simulink model "RobotX_ss_acousticsSKIP_dock_odoa_ta_1021"  (R2014a)
settings: Solver=FixedStepDiscrete  StartTime=0.0  StopTime=inf  FixedStep=.25  RelTol=1e-3
undefined symbols (not defined in the file): Com1, Com2, Com3, Com4, DiscIntNeverNeededParam, standard
libraries: xpcseriallib x42, simulink x8, slrtlib x8, speedgoatlib x2, speedgoatlib_IO102 x1
(part 13 of 19)

== system RobotX_ss_acousticsSKIP_dock_odoa_ta_1021/Main FSM/ODOA/SLAM1/Models for prediction/Model39 ==
  X : Inport
  Y : Inport  Port=2
  Psi : Inport  Port=3
  Nav Messages : Inport  Port=4
  Bus Selector : BusSelector  OutputSignals=Velocity.u,Velocity.v,Velocity.r,Port.PtThrust,Port.PtAzimuth,Stbd.StThrust,Stbd.StAzimuth
  Data Store Read : DataStoreRead  DataStoreName=noiseLevel
  Demux : Demux  Outputs=3
  Discrete-Time Integrator1 : DiscreteIntegrator  SampleTime=-1  ICPrevOutput=DiscIntNeverNeededParam  ICPrevScaledInput=DiscIntNeverNeededParam
  Dynamic Model : MATLAB Function  TreatAsAtomicUnit=on
  Mux : Mux  Inputs=3
  Mux1 : Mux  Inputs=3
  Non-Holonomic Constraint : MATLAB Function  TreatAsAtomicUnit=on
  Port Thruster Model : MATLAB Function  TreatAsAtomicUnit=on
  Stbd Thruster Model : MATLAB Function  TreatAsAtomicUnit=on
  Sum : Sum  Inputs=|++|
  enabled : Constant
  move_part : MATLAB Function  TreatAsAtomicUnit=on
  NEyaw : Outport
  wires:
  Sum/1 -> Demux/1  "Forces"
  Bus Selector/2 -> Non-Holonomic Constraint/6(v), Dynamic Model/5(v)  "<v>"
  Bus Selector/1 -> Non-Holonomic Constraint/5(u), Dynamic Model/4(u)  "<u>"
  Psi/1 -> Non-Holonomic Constraint/8(psi), Dynamic Model/6(psi)
  Demux/2 -> Dynamic Model/2(F_sway)
  Demux/3 -> Dynamic Model/3(Torque)
  Demux/1 -> Dynamic Model/1(F_surge)
  Mux/1 -> Sum/2
  Stbd Thruster Model/1(F_surge) -> Mux/1
  Stbd Thruster Model/3(Torque) -> Mux/3
  Stbd Thruster Model/2(F_sway) -> Mux/2
  Mux1/1 -> Sum/1
  Port Thruster Model/2(F_sway) -> Mux1/2
  Port Thruster Model/1(F_surge) -> Mux1/1
  Port Thruster Model/3(Torque) -> Mux1/3
  Dynamic Model/1(surgeAccel) -> Non-Holonomic Constraint/2(surgeAccel)
  Dynamic Model/2(swayAccel) -> Non-Holonomic Constraint/3(swayAccel)
  Dynamic Model/3(yawAccel) -> Non-Holonomic Constraint/4(YawAccel)
  Y/1 -> Non-Holonomic Constraint/10(Y)
  X/1 -> Non-Holonomic Constraint/9(X)
  Bus Selector/3 -> Non-Holonomic Constraint/7(gyrz)  "<r>"
  Non-Holonomic Constraint/1(NEyaw) -> NEyaw/1
  enabled/1 -> Discrete-Time Integrator1/1
  Discrete-Time Integrator1/1 -> Non-Holonomic Constraint/1(time)
  Nav Messages/1 -> Bus Selector/1
  Bus Selector/4 -> move_part/1(PtThrust)  "<PtThrust>"
  Bus Selector/5 -> move_part/2(PtAzimuth)  "<PtAzimuth>"
  Bus Selector/7 -> move_part/4(StAzimuth)  "<StAzimuth>"
  Bus Selector/6 -> move_part/3(StThrust)  "<StThrust>"
  move_part/1(portMP) -> Port Thruster Model/1(portMP)
  move_part/2(portAzimuth) -> Port Thruster Model/2(portAzimuth)
  move_part/3(stbdMP) -> Stbd Thruster Model/1(stbdMP)
  move_part/4(stbdAzimuth) -> Stbd Thruster Model/2(stbdAzimuth)
  Data Store Read/1 -> move_part/5(noiseLevel)

== system RobotX_ss_acousticsSKIP_dock_odoa_ta_1021/Main FSM/ODOA/SLAM1/Models for prediction/Model4 ==
  X : Inport
  Y : Inport  Port=2
  Psi : Inport  Port=3
  Nav Messages : Inport  Port=4
  Bus Selector : BusSelector  OutputSignals=Velocity.u,Velocity.v,Velocity.r,Port.PtThrust,Port.PtAzimuth,Stbd.StThrust,Stbd.StAzimuth
  Data Store Read : DataStoreRead  DataStoreName=noiseLevel
  Demux : Demux  Outputs=3
  Discrete-Time Integrator1 : DiscreteIntegrator  SampleTime=-1  ICPrevOutput=DiscIntNeverNeededParam  ICPrevScaledInput=DiscIntNeverNeededParam
  Dynamic Model : MATLAB Function  TreatAsAtomicUnit=on
  Mux : Mux  Inputs=3
  Mux1 : Mux  Inputs=3
  Non-Holonomic Constraint : MATLAB Function  TreatAsAtomicUnit=on
  Port Thruster Model : MATLAB Function  TreatAsAtomicUnit=on
  Stbd Thruster Model : MATLAB Function  TreatAsAtomicUnit=on
  Sum : Sum  Inputs=|++|
  enabled : Constant
  move_part : MATLAB Function  TreatAsAtomicUnit=on
  NEyaw : Outport
  wires:
  Sum/1 -> Demux/1  "Forces"
  Bus Selector/2 -> Non-Holonomic Constraint/6(v), Dynamic Model/5(v)  "<v>"
  Bus Selector/1 -> Non-Holonomic Constraint/5(u), Dynamic Model/4(u)  "<u>"
  Psi/1 -> Non-Holonomic Constraint/8(psi), Dynamic Model/6(psi)
  Demux/2 -> Dynamic Model/2(F_sway)
  Demux/3 -> Dynamic Model/3(Torque)
  Demux/1 -> Dynamic Model/1(F_surge)
  Mux/1 -> Sum/2
  Stbd Thruster Model/1(F_surge) -> Mux/1
  Stbd Thruster Model/3(Torque) -> Mux/3
  Stbd Thruster Model/2(F_sway) -> Mux/2
  Mux1/1 -> Sum/1
  Port Thruster Model/2(F_sway) -> Mux1/2
  Port Thruster Model/1(F_surge) -> Mux1/1
  Port Thruster Model/3(Torque) -> Mux1/3
  Dynamic Model/1(surgeAccel) -> Non-Holonomic Constraint/2(surgeAccel)
  Dynamic Model/2(swayAccel) -> Non-Holonomic Constraint/3(swayAccel)
  Dynamic Model/3(yawAccel) -> Non-Holonomic Constraint/4(YawAccel)
  Y/1 -> Non-Holonomic Constraint/10(Y)
  X/1 -> Non-Holonomic Constraint/9(X)
  Bus Selector/3 -> Non-Holonomic Constraint/7(gyrz)  "<r>"
  Non-Holonomic Constraint/1(NEyaw) -> NEyaw/1
  enabled/1 -> Discrete-Time Integrator1/1
  Discrete-Time Integrator1/1 -> Non-Holonomic Constraint/1(time)
  Nav Messages/1 -> Bus Selector/1
  Bus Selector/4 -> move_part/1(PtThrust)  "<PtThrust>"
  Bus Selector/5 -> move_part/2(PtAzimuth)  "<PtAzimuth>"
  Bus Selector/7 -> move_part/4(StAzimuth)  "<StAzimuth>"
  Bus Selector/6 -> move_part/3(StThrust)  "<StThrust>"
  move_part/1(portMP) -> Port Thruster Model/1(portMP)
  move_part/2(portAzimuth) -> Port Thruster Model/2(portAzimuth)
  move_part/3(stbdMP) -> Stbd Thruster Model/1(stbdMP)
  move_part/4(stbdAzimuth) -> Stbd Thruster Model/2(stbdAzimuth)
  Data Store Read/1 -> move_part/5(noiseLevel)

== system RobotX_ss_acousticsSKIP_dock_odoa_ta_1021/Main FSM/ODOA/SLAM1/Models for prediction/Model40 ==
  X : Inport
  Y : Inport  Port=2
  Psi : Inport  Port=3
  Nav Messages : Inport  Port=4
  Bus Selector : BusSelector  OutputSignals=Velocity.u,Velocity.v,Velocity.r,Port.PtThrust,Port.PtAzimuth,Stbd.StThrust,Stbd.StAzimuth
  Data Store Read : DataStoreRead  DataStoreName=noiseLevel
  Demux : Demux  Outputs=3
  Discrete-Time Integrator1 : DiscreteIntegrator  SampleTime=-1  ICPrevOutput=DiscIntNeverNeededParam  ICPrevScaledInput=DiscIntNeverNeededParam
  Dynamic Model : MATLAB Function  TreatAsAtomicUnit=on
  Mux : Mux  Inputs=3
  Mux1 : Mux  Inputs=3
  Non-Holonomic Constraint : MATLAB Function  TreatAsAtomicUnit=on
  Port Thruster Model : MATLAB Function  TreatAsAtomicUnit=on
  Stbd Thruster Model : MATLAB Function  TreatAsAtomicUnit=on
  Sum : Sum  Inputs=|++|
  enabled : Constant
  move_part : MATLAB Function  TreatAsAtomicUnit=on
  NEyaw : Outport
  wires:
  Sum/1 -> Demux/1  "Forces"
  Bus Selector/2 -> Non-Holonomic Constraint/6(v), Dynamic Model/5(v)  "<v>"
  Bus Selector/1 -> Non-Holonomic Constraint/5(u), Dynamic Model/4(u)  "<u>"
  Psi/1 -> Non-Holonomic Constraint/8(psi), Dynamic Model/6(psi)
  Demux/2 -> Dynamic Model/2(F_sway)
  Demux/3 -> Dynamic Model/3(Torque)
  Demux/1 -> Dynamic Model/1(F_surge)
  Mux/1 -> Sum/2
  Stbd Thruster Model/1(F_surge) -> Mux/1
  Stbd Thruster Model/3(Torque) -> Mux/3
  Stbd Thruster Model/2(F_sway) -> Mux/2
  Mux1/1 -> Sum/1
  Port Thruster Model/2(F_sway) -> Mux1/2
  Port Thruster Model/1(F_surge) -> Mux1/1
  Port Thruster Model/3(Torque) -> Mux1/3
  Dynamic Model/1(surgeAccel) -> Non-Holonomic Constraint/2(surgeAccel)
  Dynamic Model/2(swayAccel) -> Non-Holonomic Constraint/3(swayAccel)
  Dynamic Model/3(yawAccel) -> Non-Holonomic Constraint/4(YawAccel)
  Y/1 -> Non-Holonomic Constraint/10(Y)
  X/1 -> Non-Holonomic Constraint/9(X)
  Bus Selector/3 -> Non-Holonomic Constraint/7(gyrz)  "<r>"
  Non-Holonomic Constraint/1(NEyaw) -> NEyaw/1
  enabled/1 -> Discrete-Time Integrator1/1
  Discrete-Time Integrator1/1 -> Non-Holonomic Constraint/1(time)
  Nav Messages/1 -> Bus Selector/1
  Bus Selector/4 -> move_part/1(PtThrust)  "<PtThrust>"
  Bus Selector/5 -> move_part/2(PtAzimuth)  "<PtAzimuth>"
  Bus Selector/7 -> move_part/4(StAzimuth)  "<StAzimuth>"
  Bus Selector/6 -> move_part/3(StThrust)  "<StThrust>"
  move_part/1(portMP) -> Port Thruster Model/1(portMP)
  move_part/2(portAzimuth) -> Port Thruster Model/2(portAzimuth)
  move_part/3(stbdMP) -> Stbd Thruster Model/1(stbdMP)
  move_part/4(stbdAzimuth) -> Stbd Thruster Model/2(stbdAzimuth)
  Data Store Read/1 -> move_part/5(noiseLevel)

== system RobotX_ss_acousticsSKIP_dock_odoa_ta_1021/Main FSM/ODOA/SLAM1/Models for prediction/Model41 ==
  X : Inport
  Y : Inport  Port=2
  Psi : Inport  Port=3
  Nav Messages : Inport  Port=4
  Bus Selector : BusSelector  OutputSignals=Velocity.u,Velocity.v,Velocity.r,Port.PtThrust,Port.PtAzimuth,Stbd.StThrust,Stbd.StAzimuth
  Data Store Read : DataStoreRead  DataStoreName=noiseLevel
  Demux : Demux  Outputs=3
  Discrete-Time Integrator1 : DiscreteIntegrator  SampleTime=-1  ICPrevOutput=DiscIntNeverNeededParam  ICPrevScaledInput=DiscIntNeverNeededParam
  Dynamic Model : MATLAB Function  TreatAsAtomicUnit=on
  Mux : Mux  Inputs=3
  Mux1 : Mux  Inputs=3
  Non-Holonomic Constraint : MATLAB Function  TreatAsAtomicUnit=on
  Port Thruster Model : MATLAB Function  TreatAsAtomicUnit=on
  Stbd Thruster Model : MATLAB Function  TreatAsAtomicUnit=on
  Sum : Sum  Inputs=|++|
  enabled : Constant
  move_part : MATLAB Function  TreatAsAtomicUnit=on
  NEyaw : Outport
  wires:
  Sum/1 -> Demux/1  "Forces"
  Bus Selector/2 -> Non-Holonomic Constraint/6(v), Dynamic Model/5(v)  "<v>"
  Bus Selector/1 -> Non-Holonomic Constraint/5(u), Dynamic Model/4(u)  "<u>"
  Psi/1 -> Non-Holonomic Constraint/8(psi), Dynamic Model/6(psi)
  Demux/2 -> Dynamic Model/2(F_sway)
  Demux/3 -> Dynamic Model/3(Torque)
  Demux/1 -> Dynamic Model/1(F_surge)
  Mux/1 -> Sum/2
  Stbd Thruster Model/1(F_surge) -> Mux/1
  Stbd Thruster Model/3(Torque) -> Mux/3
  Stbd Thruster Model/2(F_sway) -> Mux/2
  Mux1/1 -> Sum/1
  Port Thruster Model/2(F_sway) -> Mux1/2
  Port Thruster Model/1(F_surge) -> Mux1/1
  Port Thruster Model/3(Torque) -> Mux1/3
  Dynamic Model/1(surgeAccel) -> Non-Holonomic Constraint/2(surgeAccel)
  Dynamic Model/2(swayAccel) -> Non-Holonomic Constraint/3(swayAccel)
  Dynamic Model/3(yawAccel) -> Non-Holonomic Constraint/4(YawAccel)
  Y/1 -> Non-Holonomic Constraint/10(Y)
  X/1 -> Non-Holonomic Constraint/9(X)
  Bus Selector/3 -> Non-Holonomic Constraint/7(gyrz)  "<r>"
  Non-Holonomic Constraint/1(NEyaw) -> NEyaw/1
  enabled/1 -> Discrete-Time Integrator1/1
  Discrete-Time Integrator1/1 -> Non-Holonomic Constraint/1(time)
  Nav Messages/1 -> Bus Selector/1
  Bus Selector/4 -> move_part/1(PtThrust)  "<PtThrust>"
  Bus Selector/5 -> move_part/2(PtAzimuth)  "<PtAzimuth>"
  Bus Selector/7 -> move_part/4(StAzimuth)  "<StAzimuth>"
  Bus Selector/6 -> move_part/3(StThrust)  "<StThrust>"
  move_part/1(portMP) -> Port Thruster Model/1(portMP)
  move_part/2(portAzimuth) -> Port Thruster Model/2(portAzimuth)
  move_part/3(stbdMP) -> Stbd Thruster Model/1(stbdMP)
  move_part/4(stbdAzimuth) -> Stbd Thruster Model/2(stbdAzimuth)
  Data Store Read/1 -> move_part/5(noiseLevel)

== system RobotX_ss_acousticsSKIP_dock_odoa_ta_1021/Main FSM/ODOA/SLAM1/Models for prediction/Model42 ==
  X : Inport
  Y : Inport  Port=2
  Psi : Inport  Port=3
  Nav Messages : Inport  Port=4
  Bus Selector : BusSelector  OutputSignals=Velocity.u,Velocity.v,Velocity.r,Port.PtThrust,Port.PtAzimuth,Stbd.StThrust,Stbd.StAzimuth
  Data Store Read : DataStoreRead  DataStoreName=noiseLevel
  Demux : Demux  Outputs=3
  Discrete-Time Integrator1 : DiscreteIntegrator  SampleTime=-1  ICPrevOutput=DiscIntNeverNeededParam  ICPrevScaledInput=DiscIntNeverNeededParam
  Dynamic Model : MATLAB Function  TreatAsAtomicUnit=on
  Mux : Mux  Inputs=3
  Mux1 : Mux  Inputs=3
  Non-Holonomic Constraint : MATLAB Function  TreatAsAtomicUnit=on
  Port Thruster Model : MATLAB Function  TreatAsAtomicUnit=on
  Stbd Thruster Model : MATLAB Function  TreatAsAtomicUnit=on
  Sum : Sum  Inputs=|++|
  enabled : Constant
  move_part : MATLAB Function  TreatAsAtomicUnit=on
  NEyaw : Outport
  wires:
  Sum/1 -> Demux/1  "Forces"
  Bus Selector/2 -> Non-Holonomic Constraint/6(v), Dynamic Model/5(v)  "<v>"
  Bus Selector/1 -> Non-Holonomic Constraint/5(u), Dynamic Model/4(u)  "<u>"
  Psi/1 -> Non-Holonomic Constraint/8(psi), Dynamic Model/6(psi)
  Demux/2 -> Dynamic Model/2(F_sway)
  Demux/3 -> Dynamic Model/3(Torque)
  Demux/1 -> Dynamic Model/1(F_surge)
  Mux/1 -> Sum/2
  Stbd Thruster Model/1(F_surge) -> Mux/1
  Stbd Thruster Model/3(Torque) -> Mux/3
  Stbd Thruster Model/2(F_sway) -> Mux/2
  Mux1/1 -> Sum/1
  Port Thruster Model/2(F_sway) -> Mux1/2
  Port Thruster Model/1(F_surge) -> Mux1/1
  Port Thruster Model/3(Torque) -> Mux1/3
  Dynamic Model/1(surgeAccel) -> Non-Holonomic Constraint/2(surgeAccel)
  Dynamic Model/2(swayAccel) -> Non-Holonomic Constraint/3(swayAccel)
  Dynamic Model/3(yawAccel) -> Non-Holonomic Constraint/4(YawAccel)
  Y/1 -> Non-Holonomic Constraint/10(Y)
  X/1 -> Non-Holonomic Constraint/9(X)
  Bus Selector/3 -> Non-Holonomic Constraint/7(gyrz)  "<r>"
  Non-Holonomic Constraint/1(NEyaw) -> NEyaw/1
  enabled/1 -> Discrete-Time Integrator1/1
  Discrete-Time Integrator1/1 -> Non-Holonomic Constraint/1(time)
  Nav Messages/1 -> Bus Selector/1
  Bus Selector/4 -> move_part/1(PtThrust)  "<PtThrust>"
  Bus Selector/5 -> move_part/2(PtAzimuth)  "<PtAzimuth>"
  Bus Selector/7 -> move_part/4(StAzimuth)  "<StAzimuth>"
  Bus Selector/6 -> move_part/3(StThrust)  "<StThrust>"
  move_part/1(portMP) -> Port Thruster Model/1(portMP)
  move_part/2(portAzimuth) -> Port Thruster Model/2(portAzimuth)
  move_part/3(stbdMP) -> Stbd Thruster Model/1(stbdMP)
  move_part/4(stbdAzimuth) -> Stbd Thruster Model/2(stbdAzimuth)
  Data Store Read/1 -> move_part/5(noiseLevel)

== system RobotX_ss_acousticsSKIP_dock_odoa_ta_1021/Main FSM/ODOA/SLAM1/Models for prediction/Model43 ==
  X : Inport
  Y : Inport  Port=2
  Psi : Inport  Port=3
  Nav Messages : Inport  Port=4
  Bus Selector : BusSelector  OutputSignals=Velocity.u,Velocity.v,Velocity.r,Port.PtThrust,Port.PtAzimuth,Stbd.StThrust,Stbd.StAzimuth
  Data Store Read : DataStoreRead  DataStoreName=noiseLevel
  Demux : Demux  Outputs=3
  Discrete-Time Integrator1 : DiscreteIntegrator  SampleTime=-1  ICPrevOutput=DiscIntNeverNeededParam  ICPrevScaledInput=DiscIntNeverNeededParam
  Dynamic Model : MATLAB Function  TreatAsAtomicUnit=on
  Mux : Mux  Inputs=3
  Mux1 : Mux  Inputs=3
  Non-Holonomic Constraint : MATLAB Function  TreatAsAtomicUnit=on
  Port Thruster Model : MATLAB Function  TreatAsAtomicUnit=on
  Stbd Thruster Model : MATLAB Function  TreatAsAtomicUnit=on
  Sum : Sum  Inputs=|++|
  enabled : Constant
  move_part : MATLAB Function  TreatAsAtomicUnit=on
  NEyaw : Outport
  wires:
  Sum/1 -> Demux/1  "Forces"
  Bus Selector/2 -> Non-Holonomic Constraint/6(v), Dynamic Model/5(v)  "<v>"
  Bus Selector/1 -> Non-Holonomic Constraint/5(u), Dynamic Model/4(u)  "<u>"
  Psi/1 -> Non-Holonomic Constraint/8(psi), Dynamic Model/6(psi)
  Demux/2 -> Dynamic Model/2(F_sway)
  Demux/3 -> Dynamic Model/3(Torque)
  Demux/1 -> Dynamic Model/1(F_surge)
  Mux/1 -> Sum/2
  Stbd Thruster Model/1(F_surge) -> Mux/1
  Stbd Thruster Model/3(Torque) -> Mux/3
  Stbd Thruster Model/2(F_sway) -> Mux/2
  Mux1/1 -> Sum/1
  Port Thruster Model/2(F_sway) -> Mux1/2
  Port Thruster Model/1(F_surge) -> Mux1/1
  Port Thruster Model/3(Torque) -> Mux1/3
  Dynamic Model/1(surgeAccel) -> Non-Holonomic Constraint/2(surgeAccel)
  Dynamic Model/2(swayAccel) -> Non-Holonomic Constraint/3(swayAccel)
  Dynamic Model/3(yawAccel) -> Non-Holonomic Constraint/4(YawAccel)
  Y/1 -> Non-Holonomic Constraint/10(Y)
  X/1 -> Non-Holonomic Constraint/9(X)
  Bus Selector/3 -> Non-Holonomic Constraint/7(gyrz)  "<r>"
  Non-Holonomic Constraint/1(NEyaw) -> NEyaw/1
  enabled/1 -> Discrete-Time Integrator1/1
  Discrete-Time Integrator1/1 -> Non-Holonomic Constraint/1(time)
  Nav Messages/1 -> Bus Selector/1
  Bus Selector/4 -> move_part/1(PtThrust)  "<PtThrust>"
  Bus Selector/5 -> move_part/2(PtAzimuth)  "<PtAzimuth>"
  Bus Selector/7 -> move_part/4(StAzimuth)  "<StAzimuth>"
  Bus Selector/6 -> move_part/3(StThrust)  "<StThrust>"
  move_part/1(portMP) -> Port Thruster Model/1(portMP)
  move_part/2(portAzimuth) -> Port Thruster Model/2(portAzimuth)
  move_part/3(stbdMP) -> Stbd Thruster Model/1(stbdMP)
  move_part/4(stbdAzimuth) -> Stbd Thruster Model/2(stbdAzimuth)
  Data Store Read/1 -> move_part/5(noiseLevel)

== system RobotX_ss_acousticsSKIP_dock_odoa_ta_1021/Main FSM/ODOA/SLAM1/Models for prediction/Model44 ==
  X : Inport
  Y : Inport  Port=2
  Psi : Inport  Port=3
  Nav Messages : Inport  Port=4
  Bus Selector : BusSelector  OutputSignals=Velocity.u,Velocity.v,Velocity.r,Port.PtThrust,Port.PtAzimuth,Stbd.StThrust,Stbd.StAzimuth
  Data Store Read : DataStoreRead  DataStoreName=noiseLevel
  Demux : Demux  Outputs=3
  Discrete-Time Integrator1 : DiscreteIntegrator  SampleTime=-1  ICPrevOutput=DiscIntNeverNeededParam  ICPrevScaledInput=DiscIntNeverNeededParam
  Dynamic Model : MATLAB Function  TreatAsAtomicUnit=on
  Mux : Mux  Inputs=3
  Mux1 : Mux  Inputs=3
  Non-Holonomic Constraint : MATLAB Function  TreatAsAtomicUnit=on
  Port Thruster Model : MATLAB Function  TreatAsAtomicUnit=on
  Stbd Thruster Model : MATLAB Function  TreatAsAtomicUnit=on
  Sum : Sum  Inputs=|++|
  enabled : Constant
  move_part : MATLAB Function  TreatAsAtomicUnit=on
  NEyaw : Outport
  wires:
  Sum/1 -> Demux/1  "Forces"
  Bus Selector/2 -> Non-Holonomic Constraint/6(v), Dynamic Model/5(v)  "<v>"
  Bus Selector/1 -> Non-Holonomic Constraint/5(u), Dynamic Model/4(u)  "<u>"
  Psi/1 -> Non-Holonomic Constraint/8(psi), Dynamic Model/6(psi)
  Demux/2 -> Dynamic Model/2(F_sway)
  Demux/3 -> Dynamic Model/3(Torque)
  Demux/1 -> Dynamic Model/1(F_surge)
  Mux/1 -> Sum/2
  Stbd Thruster Model/1(F_surge) -> Mux/1
  Stbd Thruster Model/3(Torque) -> Mux/3
  Stbd Thruster Model/2(F_sway) -> Mux/2
  Mux1/1 -> Sum/1
  Port Thruster Model/2(F_sway) -> Mux1/2
  Port Thruster Model/1(F_surge) -> Mux1/1
  Port Thruster Model/3(Torque) -> Mux1/3
  Dynamic Model/1(surgeAccel) -> Non-Holonomic Constraint/2(surgeAccel)
  Dynamic Model/2(swayAccel) -> Non-Holonomic Constraint/3(swayAccel)
  Dynamic Model/3(yawAccel) -> Non-Holonomic Constraint/4(YawAccel)
  Y/1 -> Non-Holonomic Constraint/10(Y)
  X/1 -> Non-Holonomic Constraint/9(X)
  Bus Selector/3 -> Non-Holonomic Constraint/7(gyrz)  "<r>"
  Non-Holonomic Constraint/1(NEyaw) -> NEyaw/1
  enabled/1 -> Discrete-Time Integrator1/1
  Discrete-Time Integrator1/1 -> Non-Holonomic Constraint/1(time)
  Nav Messages/1 -> Bus Selector/1
  Bus Selector/4 -> move_part/1(PtThrust)  "<PtThrust>"
  Bus Selector/5 -> move_part/2(PtAzimuth)  "<PtAzimuth>"
  Bus Selector/7 -> move_part/4(StAzimuth)  "<StAzimuth>"
  Bus Selector/6 -> move_part/3(StThrust)  "<StThrust>"
  move_part/1(portMP) -> Port Thruster Model/1(portMP)
  move_part/2(portAzimuth) -> Port Thruster Model/2(portAzimuth)
  move_part/3(stbdMP) -> Stbd Thruster Model/1(stbdMP)
  move_part/4(stbdAzimuth) -> Stbd Thruster Model/2(stbdAzimuth)
  Data Store Read/1 -> move_part/5(noiseLevel)

== system RobotX_ss_acousticsSKIP_dock_odoa_ta_1021/Main FSM/ODOA/SLAM1/Models for prediction/Model45 ==
  X : Inport
  Y : Inport  Port=2
  Psi : Inport  Port=3
  Nav Messages : Inport  Port=4
  Bus Selector : BusSelector  OutputSignals=Velocity.u,Velocity.v,Velocity.r,Port.PtThrust,Port.PtAzimuth,Stbd.StThrust,Stbd.StAzimuth
  Data Store Read : DataStoreRead  DataStoreName=noiseLevel
  Demux : Demux  Outputs=3
  Discrete-Time Integrator1 : DiscreteIntegrator  SampleTime=-1  ICPrevOutput=DiscIntNeverNeededParam  ICPrevScaledInput=DiscIntNeverNeededParam
  Dynamic Model : MATLAB Function  TreatAsAtomicUnit=on
  Mux : Mux  Inputs=3
  Mux1 : Mux  Inputs=3
  Non-Holonomic Constraint : MATLAB Function  TreatAsAtomicUnit=on
  Port Thruster Model : MATLAB Function  TreatAsAtomicUnit=on
  Stbd Thruster Model : MATLAB Function  TreatAsAtomicUnit=on
  Sum : Sum  Inputs=|++|
  enabled : Constant
  move_part : MATLAB Function  TreatAsAtomicUnit=on
  NEyaw : Outport
  wires:
  Sum/1 -> Demux/1  "Forces"
  Bus Selector/2 -> Non-Holonomic Constraint/6(v), Dynamic Model/5(v)  "<v>"
  Bus Selector/1 -> Non-Holonomic Constraint/5(u), Dynamic Model/4(u)  "<u>"
  Psi/1 -> Non-Holonomic Constraint/8(psi), Dynamic Model/6(psi)
  Demux/2 -> Dynamic Model/2(F_sway)
  Demux/3 -> Dynamic Model/3(Torque)
  Demux/1 -> Dynamic Model/1(F_surge)
  Mux/1 -> Sum/2
  Stbd Thruster Model/1(F_surge) -> Mux/1
  Stbd Thruster Model/3(Torque) -> Mux/3
  Stbd Thruster Model/2(F_sway) -> Mux/2
  Mux1/1 -> Sum/1
  Port Thruster Model/2(F_sway) -> Mux1/2
  Port Thruster Model/1(F_surge) -> Mux1/1
  Port Thruster Model/3(Torque) -> Mux1/3
  Dynamic Model/1(surgeAccel) -> Non-Holonomic Constraint/2(surgeAccel)
  Dynamic Model/2(swayAccel) -> Non-Holonomic Constraint/3(swayAccel)
  Dynamic Model/3(yawAccel) -> Non-Holonomic Constraint/4(YawAccel)
  Y/1 -> Non-Holonomic Constraint/10(Y)
  X/1 -> Non-Holonomic Constraint/9(X)
  Bus Selector/3 -> Non-Holonomic Constraint/7(gyrz)  "<r>"
  Non-Holonomic Constraint/1(NEyaw) -> NEyaw/1
  enabled/1 -> Discrete-Time Integrator1/1
  Discrete-Time Integrator1/1 -> Non-Holonomic Constraint/1(time)
  Nav Messages/1 -> Bus Selector/1
  Bus Selector/4 -> move_part/1(PtThrust)  "<PtThrust>"
  Bus Selector/5 -> move_part/2(PtAzimuth)  "<PtAzimuth>"
  Bus Selector/7 -> move_part/4(StAzimuth)  "<StAzimuth>"
  Bus Selector/6 -> move_part/3(StThrust)  "<StThrust>"
  move_part/1(portMP) -> Port Thruster Model/1(portMP)
  move_part/2(portAzimuth) -> Port Thruster Model/2(portAzimuth)
  move_part/3(stbdMP) -> Stbd Thruster Model/1(stbdMP)
  move_part/4(stbdAzimuth) -> Stbd Thruster Model/2(stbdAzimuth)
  Data Store Read/1 -> move_part/5(noiseLevel)

== system RobotX_ss_acousticsSKIP_dock_odoa_ta_1021/Main FSM/ODOA/SLAM1/Models for prediction/Model46 ==
  X : Inport
  Y : Inport  Port=2
  Psi : Inport  Port=3
  Nav Messages : Inport  Port=4
  Bus Selector : BusSelector  OutputSignals=Velocity.u,Velocity.v,Velocity.r,Port.PtThrust,Port.PtAzimuth,Stbd.StThrust,Stbd.StAzimuth
  Data Store Read : DataStoreRead  DataStoreName=noiseLevel
  Demux : Demux  Outputs=3
  Discrete-Time Integrator1 : DiscreteIntegrator  SampleTime=-1  ICPrevOutput=DiscIntNeverNeededParam  ICPrevScaledInput=DiscIntNeverNeededParam
  Dynamic Model : MATLAB Function  TreatAsAtomicUnit=on
  Mux : Mux  Inputs=3
  Mux1 : Mux  Inputs=3
  Non-Holonomic Constraint : MATLAB Function  TreatAsAtomicUnit=on
  Port Thruster Model : MATLAB Function  TreatAsAtomicUnit=on
  Stbd Thruster Model : MATLAB Function  TreatAsAtomicUnit=on
  Sum : Sum  Inputs=|++|
  enabled : Constant
  move_part : MATLAB Function  TreatAsAtomicUnit=on
  NEyaw : Outport
  wires:
  Sum/1 -> Demux/1  "Forces"
  Bus Selector/2 -> Non-Holonomic Constraint/6(v), Dynamic Model/5(v)  "<v>"
  Bus Selector/1 -> Non-Holonomic Constraint/5(u), Dynamic Model/4(u)  "<u>"
  Psi/1 -> Non-Holonomic Constraint/8(psi), Dynamic Model/6(psi)
  Demux/2 -> Dynamic Model/2(F_sway)
  Demux/3 -> Dynamic Model/3(Torque)
  Demux/1 -> Dynamic Model/1(F_surge)
  Mux/1 -> Sum/2
  Stbd Thruster Model/1(F_surge) -> Mux/1
  Stbd Thruster Model/3(Torque) -> Mux/3
  Stbd Thruster Model/2(F_sway) -> Mux/2
  Mux1/1 -> Sum/1
  Port Thruster Model/2(F_sway) -> Mux1/2
  Port Thruster Model/1(F_surge) -> Mux1/1
  Port Thruster Model/3(Torque) -> Mux1/3
  Dynamic Model/1(surgeAccel) -> Non-Holonomic Constraint/2(surgeAccel)
  Dynamic Model/2(swayAccel) -> Non-Holonomic Constraint/3(swayAccel)
  Dynamic Model/3(yawAccel) -> Non-Holonomic Constraint/4(YawAccel)
  Y/1 -> Non-Holonomic Constraint/10(Y)
  X/1 -> Non-Holonomic Constraint/9(X)
  Bus Selector/3 -> Non-Holonomic Constraint/7(gyrz)  "<r>"
  Non-Holonomic Constraint/1(NEyaw) -> NEyaw/1
  enabled/1 -> Discrete-Time Integrator1/1
  Discrete-Time Integrator1/1 -> Non-Holonomic Constraint/1(time)
  Nav Messages/1 -> Bus Selector/1
  Bus Selector/4 -> move_part/1(PtThrust)  "<PtThrust>"
  Bus Selector/5 -> move_part/2(PtAzimuth)  "<PtAzimuth>"
  Bus Selector/7 -> move_part/4(StAzimuth)  "<StAzimuth>"
  Bus Selector/6 -> move_part/3(StThrust)  "<StThrust>"
  move_part/1(portMP) -> Port Thruster Model/1(portMP)
  move_part/2(portAzimuth) -> Port Thruster Model/2(portAzimuth)
  move_part/3(stbdMP) -> Stbd Thruster Model/1(stbdMP)
  move_part/4(stbdAzimuth) -> Stbd Thruster Model/2(stbdAzimuth)
  Data Store Read/1 -> move_part/5(noiseLevel)

== system RobotX_ss_acousticsSKIP_dock_odoa_ta_1021/Main FSM/ODOA/SLAM1/Models for prediction/Model47 ==
  X : Inport
  Y : Inport  Port=2
  Psi : Inport  Port=3
  Nav Messages : Inport  Port=4
  Bus Selector : BusSelector  OutputSignals=Velocity.u,Velocity.v,Velocity.r,Port.PtThrust,Port.PtAzimuth,Stbd.StThrust,Stbd.StAzimuth
  Data Store Read : DataStoreRead  DataStoreName=noiseLevel
  Demux : Demux  Outputs=3
  Discrete-Time Integrator1 : DiscreteIntegrator  SampleTime=-1  ICPrevOutput=DiscIntNeverNeededParam  ICPrevScaledInput=DiscIntNeverNeededParam
  Dynamic Model : MATLAB Function  TreatAsAtomicUnit=on
  Mux : Mux  Inputs=3
  Mux1 : Mux  Inputs=3
  Non-Holonomic Constraint : MATLAB Function  TreatAsAtomicUnit=on
  Port Thruster Model : MATLAB Function  TreatAsAtomicUnit=on
  Stbd Thruster Model : MATLAB Function  TreatAsAtomicUnit=on
  Sum : Sum  Inputs=|++|
  enabled : Constant
  move_part : MATLAB Function  TreatAsAtomicUnit=on
  NEyaw : Outport
  wires:
  Sum/1 -> Demux/1  "Forces"
  Bus Selector/2 -> Non-Holonomic Constraint/6(v), Dynamic Model/5(v)  "<v>"
  Bus Selector/1 -> Non-Holonomic Constraint/5(u), Dynamic Model/4(u)  "<u>"
  Psi/1 -> Non-Holonomic Constraint/8(psi), Dynamic Model/6(psi)
  Demux/2 -> Dynamic Model/2(F_sway)
  Demux/3 -> Dynamic Model/3(Torque)
  Demux/1 -> Dynamic Model/1(F_surge)
  Mux/1 -> Sum/2
  Stbd Thruster Model/1(F_surge) -> Mux/1
  Stbd Thruster Model/3(Torque) -> Mux/3
  Stbd Thruster Model/2(F_sway) -> Mux/2
  Mux1/1 -> Sum/1
  Port Thruster Model/2(F_sway) -> Mux1/2
  Port Thruster Model/1(F_surge) -> Mux1/1
  Port Thruster Model/3(Torque) -> Mux1/3
  Dynamic Model/1(surgeAccel) -> Non-Holonomic Constraint/2(surgeAccel)
  Dynamic Model/2(swayAccel) -> Non-Holonomic Constraint/3(swayAccel)
  Dynamic Model/3(yawAccel) -> Non-Holonomic Constraint/4(YawAccel)
  Y/1 -> Non-Holonomic Constraint/10(Y)
  X/1 -> Non-Holonomic Constraint/9(X)
  Bus Selector/3 -> Non-Holonomic Constraint/7(gyrz)  "<r>"
  Non-Holonomic Constraint/1(NEyaw) -> NEyaw/1
  enabled/1 -> Discrete-Time Integrator1/1
  Discrete-Time Integrator1/1 -> Non-Holonomic Constraint/1(time)
  Nav Messages/1 -> Bus Selector/1
  Bus Selector/4 -> move_part/1(PtThrust)  "<PtThrust>"
  Bus Selector/5 -> move_part/2(PtAzimuth)  "<PtAzimuth>"
  Bus Selector/7 -> move_part/4(StAzimuth)  "<StAzimuth>"
  Bus Selector/6 -> move_part/3(StThrust)  "<StThrust>"
  move_part/1(portMP) -> Port Thruster Model/1(portMP)
  move_part/2(portAzimuth) -> Port Thruster Model/2(portAzimuth)
  move_part/3(stbdMP) -> Stbd Thruster Model/1(stbdMP)
  move_part/4(stbdAzimuth) -> Stbd Thruster Model/2(stbdAzimuth)
  Data Store Read/1 -> move_part/5(noiseLevel)

== system RobotX_ss_acousticsSKIP_dock_odoa_ta_1021/Main FSM/ODOA/SLAM1/Models for prediction/Model48 ==
  X : Inport
  Y : Inport  Port=2
  Psi : Inport  Port=3
  Nav Messages : Inport  Port=4
  Bus Selector : BusSelector  OutputSignals=Velocity.u,Velocity.v,Velocity.r,Port.PtThrust,Port.PtAzimuth,Stbd.StThrust,Stbd.StAzimuth
  Data Store Read : DataStoreRead  DataStoreName=noiseLevel
  Demux : Demux  Outputs=3
  Discrete-Time Integrator1 : DiscreteIntegrator  SampleTime=-1  ICPrevOutput=DiscIntNeverNeededParam  ICPrevScaledInput=DiscIntNeverNeededParam
  Dynamic Model : MATLAB Function  TreatAsAtomicUnit=on
  Mux : Mux  Inputs=3
  Mux1 : Mux  Inputs=3
  Non-Holonomic Constraint : MATLAB Function  TreatAsAtomicUnit=on
  Port Thruster Model : MATLAB Function  TreatAsAtomicUnit=on
  Stbd Thruster Model : MATLAB Function  TreatAsAtomicUnit=on
  Sum : Sum  Inputs=|++|
  enabled : Constant
  move_part : MATLAB Function  TreatAsAtomicUnit=on
  NEyaw : Outport
  wires:
  Sum/1 -> Demux/1  "Forces"
  Bus Selector/2 -> Non-Holonomic Constraint/6(v), Dynamic Model/5(v)  "<v>"
  Bus Selector/1 -> Non-Holonomic Constraint/5(u), Dynamic Model/4(u)  "<u>"
  Psi/1 -> Non-Holonomic Constraint/8(psi), Dynamic Model/6(psi)
  Demux/2 -> Dynamic Model/2(F_sway)
  Demux/3 -> Dynamic Model/3(Torque)
  Demux/1 -> Dynamic Model/1(F_surge)
  Mux/1 -> Sum/2
  Stbd Thruster Model/1(F_surge) -> Mux/1
  Stbd Thruster Model/3(Torque) -> Mux/3
  Stbd Thruster Model/2(F_sway) -> Mux/2
  Mux1/1 -> Sum/1
  Port Thruster Model/2(F_sway) -> Mux1/2
  Port Thruster Model/1(F_surge) -> Mux1/1
  Port Thruster Model/3(Torque) -> Mux1/3
  Dynamic Model/1(surgeAccel) -> Non-Holonomic Constraint/2(surgeAccel)
  Dynamic Model/2(swayAccel) -> Non-Holonomic Constraint/3(swayAccel)
  Dynamic Model/3(yawAccel) -> Non-Holonomic Constraint/4(YawAccel)
  Y/1 -> Non-Holonomic Constraint/10(Y)
  X/1 -> Non-Holonomic Constraint/9(X)
  Bus Selector/3 -> Non-Holonomic Constraint/7(gyrz)  "<r>"
  Non-Holonomic Constraint/1(NEyaw) -> NEyaw/1
  enabled/1 -> Discrete-Time Integrator1/1
  Discrete-Time Integrator1/1 -> Non-Holonomic Constraint/1(time)
  Nav Messages/1 -> Bus Selector/1
  Bus Selector/4 -> move_part/1(PtThrust)  "<PtThrust>"
  Bus Selector/5 -> move_part/2(PtAzimuth)  "<PtAzimuth>"
  Bus Selector/7 -> move_part/4(StAzimuth)  "<StAzimuth>"
  Bus Selector/6 -> move_part/3(StThrust)  "<StThrust>"
  move_part/1(portMP) -> Port Thruster Model/1(portMP)
  move_part/2(portAzimuth) -> Port Thruster Model/2(portAzimuth)
  move_part/3(stbdMP) -> Stbd Thruster Model/1(stbdMP)
  move_part/4(stbdAzimuth) -> Stbd Thruster Model/2(stbdAzimuth)
  Data Store Read/1 -> move_part/5(noiseLevel)

== system RobotX_ss_acousticsSKIP_dock_odoa_ta_1021/Main FSM/ODOA/SLAM1/Models for prediction/Model49 ==
  X : Inport
  Y : Inport  Port=2
  Psi : Inport  Port=3
  Nav Messages : Inport  Port=4
  Bus Selector : BusSelector  OutputSignals=Velocity.u,Velocity.v,Velocity.r,Port.PtThrust,Port.PtAzimuth,Stbd.StThrust,Stbd.StAzimuth
  Data Store Read : DataStoreRead  DataStoreName=noiseLevel
  Demux : Demux  Outputs=3
  Discrete-Time Integrator1 : DiscreteIntegrator  SampleTime=-1  ICPrevOutput=DiscIntNeverNeededParam  ICPrevScaledInput=DiscIntNeverNeededParam
  Dynamic Model : MATLAB Function  TreatAsAtomicUnit=on
  Mux : Mux  Inputs=3
  Mux1 : Mux  Inputs=3
  Non-Holonomic Constraint : MATLAB Function  TreatAsAtomicUnit=on
  Port Thruster Model : MATLAB Function  TreatAsAtomicUnit=on
  Stbd Thruster Model : MATLAB Function  TreatAsAtomicUnit=on
  Sum : Sum  Inputs=|++|
  enabled : Constant
  move_part : MATLAB Function  TreatAsAtomicUnit=on
  NEyaw : Outport
  wires:
  Sum/1 -> Demux/1  "Forces"
  Bus Selector/2 -> Non-Holonomic Constraint/6(v), Dynamic Model/5(v)  "<v>"
  Bus Selector/1 -> Non-Holonomic Constraint/5(u), Dynamic Model/4(u)  "<u>"
  Psi/1 -> Non-Holonomic Constraint/8(psi), Dynamic Model/6(psi)
  Demux/2 -> Dynamic Model/2(F_sway)
  Demux/3 -> Dynamic Model/3(Torque)
  Demux/1 -> Dynamic Model/1(F_surge)
  Mux/1 -> Sum/2
  Stbd Thruster Model/1(F_surge) -> Mux/1
  Stbd Thruster Model/3(Torque) -> Mux/3
  Stbd Thruster Model/2(F_sway) -> Mux/2
  Mux1/1 -> Sum/1
  Port Thruster Model/2(F_sway) -> Mux1/2
  Port Thruster Model/1(F_surge) -> Mux1/1
  Port Thruster Model/3(Torque) -> Mux1/3
  Dynamic Model/1(surgeAccel) -> Non-Holonomic Constraint/2(surgeAccel)
  Dynamic Model/2(swayAccel) -> Non-Holonomic Constraint/3(swayAccel)
  Dynamic Model/3(yawAccel) -> Non-Holonomic Constraint/4(YawAccel)
  Y/1 -> Non-Holonomic Constraint/10(Y)
  X/1 -> Non-Holonomic Constraint/9(X)
  Bus Selector/3 -> Non-Holonomic Constraint/7(gyrz)  "<r>"
  Non-Holonomic Constraint/1(NEyaw) -> NEyaw/1
  enabled/1 -> Discrete-Time Integrator1/1
  Discrete-Time Integrator1/1 -> Non-Holonomic Constraint/1(time)
  Nav Messages/1 -> Bus Selector/1
  Bus Selector/4 -> move_part/1(PtThrust)  "<PtThrust>"
  Bus Selector/5 -> move_part/2(PtAzimuth)  "<PtAzimuth>"
  Bus Selector/7 -> move_part/4(StAzimuth)  "<StAzimuth>"
  Bus Selector/6 -> move_part/3(StThrust)  "<StThrust>"
  move_part/1(portMP) -> Port Thruster Model/1(portMP)
  move_part/2(portAzimuth) -> Port Thruster Model/2(portAzimuth)
  move_part/3(stbdMP) -> Stbd Thruster Model/1(stbdMP)
  move_part/4(stbdAzimuth) -> Stbd Thruster Model/2(stbdAzimuth)
  Data Store Read/1 -> move_part/5(noiseLevel)

== system RobotX_ss_acousticsSKIP_dock_odoa_ta_1021/Main FSM/ODOA/SLAM1/Models for prediction/Model5 ==
  X : Inport
  Y : Inport  Port=2
  Psi : Inport  Port=3
  Nav Messages : Inport  Port=4
  Bus Selector : BusSelector  OutputSignals=Velocity.u,Velocity.v,Velocity.r,Port.PtThrust,Port.PtAzimuth,Stbd.StThrust,Stbd.StAzimuth
  Data Store Read : DataStoreRead  DataStoreName=noiseLevel
  Demux : Demux  Outputs=3
  Discrete-Time Integrator1 : DiscreteIntegrator  SampleTime=-1  ICPrevOutput=DiscIntNeverNeededParam  ICPrevScaledInput=DiscIntNeverNeededParam
  Dynamic Model : MATLAB Function  TreatAsAtomicUnit=on
  Mux : Mux  Inputs=3
  Mux1 : Mux  Inputs=3
  Non-Holonomic Constraint : MATLAB Function  TreatAsAtomicUnit=on
  Port Thruster Model : MATLAB Function  TreatAsAtomicUnit=on
  Stbd Thruster Model : MATLAB Function  TreatAsAtomicUnit=on
  Sum : Sum  Inputs=|++|
  enabled : Constant
  move_part : MATLAB Function  TreatAsAtomicUnit=on
  NEyaw : Outport
  wires:
  Sum/1 -> Demux/1  "Forces"
  Bus Selector/2 -> Non-Holonomic Constraint/6(v), Dynamic Model/5(v)  "<v>"
  Bus Selector/1 -> Non-Holonomic Constraint/5(u), Dynamic Model/4(u)  "<u>"
  Psi/1 -> Non-Holonomic Constraint/8(psi), Dynamic Model/6(psi)
  Demux/2 -> Dynamic Model/2(F_sway)
  Demux/3 -> Dynamic Model/3(Torque)
  Demux/1 -> Dynamic Model/1(F_surge)
  Mux/1 -> Sum/2
  Stbd Thruster Model/1(F_surge) -> Mux/1
  Stbd Thruster Model/3(Torque) -> Mux/3
  Stbd Thruster Model/2(F_sway) -> Mux/2
  Mux1/1 -> Sum/1
  Port Thruster Model/2(F_sway) -> Mux1/2
  Port Thruster Model/1(F_surge) -> Mux1/1
  Port Thruster Model/3(Torque) -> Mux1/3
  Dynamic Model/1(surgeAccel) -> Non-Holonomic Constraint/2(surgeAccel)
  Dynamic Model/2(swayAccel) -> Non-Holonomic Constraint/3(swayAccel)
  Dynamic Model/3(yawAccel) -> Non-Holonomic Constraint/4(YawAccel)
  Y/1 -> Non-Holonomic Constraint/10(Y)
  X/1 -> Non-Holonomic Constraint/9(X)
  Bus Selector/3 -> Non-Holonomic Constraint/7(gyrz)  "<r>"
  Non-Holonomic Constraint/1(NEyaw) -> NEyaw/1
  enabled/1 -> Discrete-Time Integrator1/1
  Discrete-Time Integrator1/1 -> Non-Holonomic Constraint/1(time)
  Nav Messages/1 -> Bus Selector/1
  Bus Selector/4 -> move_part/1(PtThrust)  "<PtThrust>"
  Bus Selector/5 -> move_part/2(PtAzimuth)  "<PtAzimuth>"
  Bus Selector/7 -> move_part/4(StAzimuth)  "<StAzimuth>"
  Bus Selector/6 -> move_part/3(StThrust)  "<StThrust>"
  move_part/1(portMP) -> Port Thruster Model/1(portMP)
  move_part/2(portAzimuth) -> Port Thruster Model/2(portAzimuth)
  move_part/3(stbdMP) -> Stbd Thruster Model/1(stbdMP)
  move_part/4(stbdAzimuth) -> Stbd Thruster Model/2(stbdAzimuth)
  Data Store Read/1 -> move_part/5(noiseLevel)

== system RobotX_ss_acousticsSKIP_dock_odoa_ta_1021/Main FSM/ODOA/SLAM1/Models for prediction/Model50 ==
  X : Inport
  Y : Inport  Port=2
  Psi : Inport  Port=3
  Nav Messages : Inport  Port=4
  Bus Selector : BusSelector  OutputSignals=Velocity.u,Velocity.v,Velocity.r,Port.PtThrust,Port.PtAzimuth,Stbd.StThrust,Stbd.StAzimuth
  Data Store Read : DataStoreRead  DataStoreName=noiseLevel
  Demux : Demux  Outputs=3
  Discrete-Time Integrator1 : DiscreteIntegrator  SampleTime=-1  ICPrevOutput=DiscIntNeverNeededParam  ICPrevScaledInput=DiscIntNeverNeededParam
  Dynamic Model : MATLAB Function  TreatAsAtomicUnit=on
  Mux : Mux  Inputs=3
  Mux1 : Mux  Inputs=3
  Non-Holonomic Constraint : MATLAB Function  TreatAsAtomicUnit=on
  Port Thruster Model : MATLAB Function  TreatAsAtomicUnit=on
  Stbd Thruster Model : MATLAB Function  TreatAsAtomicUnit=on
  Sum : Sum  Inputs=|++|
  enabled : Constant
  move_part : MATLAB Function  TreatAsAtomicUnit=on
  NEyaw : Outport
  wires:
  Sum/1 -> Demux/1  "Forces"
  Bus Selector/2 -> Non-Holonomic Constraint/6(v), Dynamic Model/5(v)  "<v>"
  Bus Selector/1 -> Non-Holonomic Constraint/5(u), Dynamic Model/4(u)  "<u>"
  Psi/1 -> Non-Holonomic Constraint/8(psi), Dynamic Model/6(psi)
  Demux/2 -> Dynamic Model/2(F_sway)
  Demux/3 -> Dynamic Model/3(Torque)
  Demux/1 -> Dynamic Model/1(F_surge)
  Mux/1 -> Sum/2
  Stbd Thruster Model/1(F_surge) -> Mux/1
  Stbd Thruster Model/3(Torque) -> Mux/3
  Stbd Thruster Model/2(F_sway) -> Mux/2
  Mux1/1 -> Sum/1
  Port Thruster Model/2(F_sway) -> Mux1/2
  Port Thruster Model/1(F_surge) -> Mux1/1
  Port Thruster Model/3(Torque) -> Mux1/3
  Dynamic Model/1(surgeAccel) -> Non-Holonomic Constraint/2(surgeAccel)
  Dynamic Model/2(swayAccel) -> Non-Holonomic Constraint/3(swayAccel)
  Dynamic Model/3(yawAccel) -> Non-Holonomic Constraint/4(YawAccel)
  Y/1 -> Non-Holonomic Constraint/10(Y)
  X/1 -> Non-Holonomic Constraint/9(X)
  Bus Selector/3 -> Non-Holonomic Constraint/7(gyrz)  "<r>"
  Non-Holonomic Constraint/1(NEyaw) -> NEyaw/1
  enabled/1 -> Discrete-Time Integrator1/1
  Discrete-Time Integrator1/1 -> Non-Holonomic Constraint/1(time)
  Nav Messages/1 -> Bus Selector/1
  Bus Selector/4 -> move_part/1(PtThrust)  "<PtThrust>"
  Bus Selector/5 -> move_part/2(PtAzimuth)  "<PtAzimuth>"
  Bus Selector/7 -> move_part/4(StAzimuth)  "<StAzimuth>"
  Bus Selector/6 -> move_part/3(StThrust)  "<StThrust>"
  move_part/1(portMP) -> Port Thruster Model/1(portMP)
  move_part/2(portAzimuth) -> Port Thruster Model/2(portAzimuth)
  move_part/3(stbdMP) -> Stbd Thruster Model/1(stbdMP)
  move_part/4(stbdAzimuth) -> Stbd Thruster Model/2(stbdAzimuth)
  Data Store Read/1 -> move_part/5(noiseLevel)

== system RobotX_ss_acousticsSKIP_dock_odoa_ta_1021/Main FSM/ODOA/SLAM1/Models for prediction/Model6 ==
  X : Inport
  Y : Inport  Port=2
  Psi : Inport  Port=3
  Nav Messages : Inport  Port=4
  Bus Selector : BusSelector  OutputSignals=Velocity.u,Velocity.v,Velocity.r,Port.PtThrust,Port.PtAzimuth,Stbd.StThrust,Stbd.StAzimuth
  Data Store Read : DataStoreRead  DataStoreName=noiseLevel
  Demux : Demux  Outputs=3
  Discrete-Time Integrator1 : DiscreteIntegrator  SampleTime=-1  ICPrevOutput=DiscIntNeverNeededParam  ICPrevScaledInput=DiscIntNeverNeededParam
  Dynamic Model : MATLAB Function  TreatAsAtomicUnit=on
  Mux : Mux  Inputs=3
  Mux1 : Mux  Inputs=3
  Non-Holonomic Constraint : MATLAB Function  TreatAsAtomicUnit=on
  Port Thruster Model : MATLAB Function  TreatAsAtomicUnit=on
  Stbd Thruster Model : MATLAB Function  TreatAsAtomicUnit=on
  Sum : Sum  Inputs=|++|
  enabled : Constant
  move_part : MATLAB Function  TreatAsAtomicUnit=on
  NEyaw : Outport
  wires:
  Sum/1 -> Demux/1  "Forces"
  Bus Selector/2 -> Non-Holonomic Constraint/6(v), Dynamic Model/5(v)  "<v>"
  Bus Selector/1 -> Non-Holonomic Constraint/5(u), Dynamic Model/4(u)  "<u>"
  Psi/1 -> Non-Holonomic Constraint/8(psi), Dynamic Model/6(psi)
  Demux/2 -> Dynamic Model/2(F_sway)
  Demux/3 -> Dynamic Model/3(Torque)
  Demux/1 -> Dynamic Model/1(F_surge)
  Mux/1 -> Sum/2
  Stbd Thruster Model/1(F_surge) -> Mux/1
  Stbd Thruster Model/3(Torque) -> Mux/3
  Stbd Thruster Model/2(F_sway) -> Mux/2
  Mux1/1 -> Sum/1
  Port Thruster Model/2(F_sway) -> Mux1/2
  Port Thruster Model/1(F_surge) -> Mux1/1
  Port Thruster Model/3(Torque) -> Mux1/3
  Dynamic Model/1(surgeAccel) -> Non-Holonomic Constraint/2(surgeAccel)
  Dynamic Model/2(swayAccel) -> Non-Holonomic Constraint/3(swayAccel)
  Dynamic Model/3(yawAccel) -> Non-Holonomic Constraint/4(YawAccel)
  Y/1 -> Non-Holonomic Constraint/10(Y)
  X/1 -> Non-Holonomic Constraint/9(X)
  Bus Selector/3 -> Non-Holonomic Constraint/7(gyrz)  "<r>"
  Non-Holonomic Constraint/1(NEyaw) -> NEyaw/1
  enabled/1 -> Discrete-Time Integrator1/1
  Discrete-Time Integrator1/1 -> Non-Holonomic Constraint/1(time)
  Nav Messages/1 -> Bus Selector/1
  Bus Selector/4 -> move_part/1(PtThrust)  "<PtThrust>"
  Bus Selector/5 -> move_part/2(PtAzimuth)  "<PtAzimuth>"
  Bus Selector/7 -> move_part/4(StAzimuth)  "<StAzimuth>"
  Bus Selector/6 -> move_part/3(StThrust)  "<StThrust>"
  move_part/1(portMP) -> Port Thruster Model/1(portMP)
  move_part/2(portAzimuth) -> Port Thruster Model/2(portAzimuth)
  move_part/3(stbdMP) -> Stbd Thruster Model/1(stbdMP)
  move_part/4(stbdAzimuth) -> Stbd Thruster Model/2(stbdAzimuth)
  Data Store Read/1 -> move_part/5(noiseLevel)

== matlab function RobotX_ss_acousticsSKIP_dock_odoa_ta_1021/Sensors/1021 Comms/Pi Nav Send/Data Update1 ==
  data: Valid input; ControlMode input; V output; C output; L output; A output; Data input; D1 output; D2 output; D3 output; D4 output; D5 output; D6 output; D7 output; D8 output; D9 output; D10 output; D11 output; D12 output; D13 output; D14 output; D15 output; D16 output; D17 output; D18 output; D19 output; D20 output; D21 output; D22 output; D23 output; D24 output; Activate input
function [V,C,L,A,D1,D2,D3,D4,D5,D6,D7,D8,D9,D10,D11,D12,D13,D14,D15,D16,D17,...
    D18,D19,D20,D21,D22,D23,D24] = dataSplit(Valid,ControlMode,Data,Activate)
%Written by Anderson Lebbad on August 10, 2014
%Last Edited by: Anderson Lebbad on September 11, 2014

%This function splits the data vector into the twelve channels it is
%composed of for communication

persistent HoldData

A = Activate;

if isempty(HoldData)
    HoldData = zeros(26,1);
end

L = 8;

if Valid == 1
    HoldData(1) = Valid;
    HoldData(2) = ControlMode;
    HoldData(3) = Data(1);
    HoldData(4) = Data(2);
    HoldData(5) = Data(3);
    HoldData(6) = Data(4);
    HoldData(7) = Data(5);
    HoldData(8) = Data(6);
    HoldData(9) = Data(7);
    HoldData(10) = Data(8);
    HoldData(11) = Data(9);
    HoldData(12) = Data(10);
    HoldData(13) = Data(11);
    HoldData(14) = Data(12);
    HoldData(15) = Data(13);
    HoldData(16) = Data(14);
    HoldData(17) = Data(15);
    HoldData(18) = Data(16);
    HoldData(19) = Data(17);
    HoldData(20) = Data(18);
    HoldData(21) = Data(19);
    HoldData(22) = Data(20);
    HoldData(23) = Data(21);
    HoldData(24) = Data(22);
    HoldData(25) = Data(23);
    HoldData(26) = Data(24);
end

V = HoldData(1);
C = HoldData(2);
D1 = HoldData(3);
D2 = HoldData(4);
D3 = HoldData(5);
D4 = HoldData(6);
D5 = HoldData(7);
D6 = HoldData(8);
D7 = HoldData(9);
D8 = HoldData(10);
D9 = HoldData(11);
D10 = HoldData(12);
D11 = HoldData(13);
D12 = HoldData(14);
D13 = HoldData(15);
D14 = HoldData(16);
D15 = HoldData(17);
D16 = HoldData(18);
D17 = HoldData(19);
D18 = HoldData(20);
D19 = HoldData(21);
D20 = HoldData(22);
D21 = HoldData(23);
D22 = HoldData(24);
D23 = HoldData(25);
D24 = HoldData(26);

end

== matlab function RobotX_ss_acousticsSKIP_dock_odoa_ta_1021/Sensors/1021 Comms/Message Selector/HRTSEA Message/MATLAB Function1 ==
  data: pingerInfo input; SEAValid output; SEALat output; SEALong output; SEAColor output; SEADepth output
function [SEAValid,SEALat,SEALong,SEAColor,SEADepth] = pingerInfoParse(pingerInfo)

SEAValid = pingerInfo(1);
SEALat = pingerInfo(2);
SEALong = pingerInfo(3);
SEADepth = pingerInfo(4);
SEAColor = pingerInfo(5);

== matlab function RobotX_ss_acousticsSKIP_dock_odoa_ta_1021/Main FSM/Docking/Dock Enabler ==
  data: taskSelector output; GpsEn output; DockEn output; ReverseEn output; mainTask input; GpsFin input; DockFin input
function [taskSelector,GpsEn,DockEn,ReverseEn]=Dock_Enabler(mainTask,GpsFin,DockFin)
%Written by Anderson Lebbad on July 19, 2013
%Last Edited: Dylan DeGaetano on September ,4 2014
%   Substring search for task was written in
%   Case switches were redundant, combined with first set of if statements

%Changes the value of MainMode and the enablers for the tasks within the
%Main FSM.

% Initialize enable signals
GpsEn = 0;
DockEn = 0;
ReverseEn = 0;

% Convert main task indicator to a string
mainTaskStr = char(mainTask);

% Adjust finished states based on user task selection (never skips
% initialization)
if ~isempty(strfind(mainTaskStr,'Dock'))
    GpsFin = 1;
elseif ~isempty(strfind(mainTaskStr,'reverse'))
    GpsFin = 1;
    DockFin = 1;
end

% Set enable signals based on state completion
if GpsFin == 0
    GpsEn = 1;
    taskSelector = 1;
elseif DockFin == 0
    DockEn = 1;
    taskSelector = 2;
else
    ReverseEn = 1 ;
    taskSelector = 3;
end

== matlab function RobotX_ss_acousticsSKIP_dock_odoa_ta_1021/Main FSM/Docking/Docking/MATLAB Function ==
  data: QuayHeading input; TargetPoint input; Finished output; X input; Data output; Y input; Psi input; Dist input; Angles input; Prob input
function [Finished,Data] = Orient(QuayHeading,TargetPoint,X,Y,Psi,Dist,Angles,Prob)
%Written by Dylan DeGaetano on September 2, 2014
%Last Edited By Anderson Lebbad on September 19 2014

%This function passes the current pose data with the requrested heading
%so that the boat is facing the Quay wall.This task must be in station
%keeping mode
%
%Anderson's edit moved the orient within this function and adjusts the code
%to work better with sensing information

%work aound for communication issue
idx = Prob(4);

persistent holdPose found

if isempty(holdPose)
    holdPose = [TargetPoint QuayHeading];
    found = 0;
end

DistM=Dist(1)/100;
Finished = 0;

%Initialize Data variable
Data = zeros(24,1);

if found == 0
    if idx(1) ~= 0
        %Calculate the NED coordinate of the found symbol
        TargetX = X+DistM(idx(1))*cos((Psi+Angles(idx(1)))*pi/180);
        TargetY = Y+DistM(idx(1))*sin((Psi+Angles(idx(1)))*pi/180);
        %Set destination in front of dock to line up
        holdPose(1) = TargetX - 10*cos(QuayHeading*pi/180);
        holdPose(2) = TargetY - 10*sin(QuayHeading*pi/180);
        holdPose(3) = QuayHeading;
        %Track that the symbol has been found
        found = 1;
    end
else
    l1norm = abs(X-holdPose(1))+abs(Y-holdPose(2));
    if l1norm < 2
        %
        holdPose(1) = holdPose(1) + 5*cos(QuayHeading*pi/180);
        holdPose(2) = holdPose(2) + 5*sin(QuayHeading*pi/180);
        found = found + 1;
    end
end

if found >= 2
    holdPose = [X Y QuayHeading];
    Finished = 1;
end

Data(1) = holdPose(1);
Data(2) = holdPose(2);
Data(3) = holdPose(3);

== matlab function RobotX_ss_acousticsSKIP_dock_odoa_ta_1021/Sensors/1020 Comms/MATLAB Function2 ==
  data: Time input; asciiLIT output; Sequence input
% This function creates the light tower message to be sent from 
% Speedgoat in ascii code
% Written by: Edward Zhu
% Date: 9/17/14

function asciiLIT = asciiLITEncoder(Time, Sequence)

% Initialize output message vector as the serial output block expects 128
% character message
asciiLIT = uint8(zeros(1,128));

% Convert static strings to ascii code
asciiMsgID = uint8('$RXLIT,');
asciiComma = uint8(',');
asciiTeamID = uint8('FAUVU,');
asciiMsgEnd = uint8('*');
asciiMsgCRLF = [13 10];

% Convert UTC Time input (hhmmss) into ascii code
asciiTime = uint8(zeros(1,7));
asciiTime(7) = asciiComma;

for timeChar = 1:6
    asciiTime(timeChar) = floor(mod(Time,10^(7-timeChar))/...
        10^(6-timeChar)) + 48;
end

% Convert the light sequece into ascii code (1 = R, 2 = B, 3 = G)
asciiSeq = uint8(zeros(1,4)+32);
asciiSeq(4) = asciiMsgEnd;

if Sequence(1) > 0 && Sequence(2) > 0 && Sequence(3) > 0
    for seqChar = 1:3
        if Sequence(seqChar) == 1
            Sequence(seqChar) = uint8('R');
        elseif Sequence(seqChar) == 2
            Sequence(seqChar) = uint8('B');
        elseif Sequence(seqChar) == 3
            Sequence(seqChar) = uint8('G');
        end
    end
    asciiSeq(1:3) = Sequence;
end

% Concat individual ascii arrays into one array
asciiPreChkSum = cat(2,asciiMsgID,asciiTime,asciiTeamID,asciiSeq);

% Calculate the checksum of the message from the '$' to the '*' and convert
% to hex
chkSum = uint8(0);

for chksumChar = 1:(length(asciiPreChkSum)-2)
    chkSum = bitxor(chkSum,asciiPreChkSum(chksumChar+1));
end

% Convert the checksum to ascii
chkSum = dec2hex(chkSum);
asciiChkSum = uint8(zeros(1,length(chkSum))+32);
for i = 1:length(chkSum)
    asciiChkSum(i) = uint8(chkSum(i));
end

% Concat the checksum and the '/r/n' to the end of the message
asciiPostChkSum = cat(2,asciiPreChkSum,asciiChkSum,asciiMsgCRLF);

% Output the final message
asciiLIT(1:length(asciiPostChkSum)) = asciiPostChkSum;

== matlab function RobotX_ss_acousticsSKIP_dock_odoa_ta_1021/Main FSM/ODOA/SLAM1/Models for prediction/Model10/move_part ==
  data: PtThrust input; portMP output; PtAzimuth input; StThrust input; StAzimuth input; noiseLevel input; portAzimuth output; stbdMP output; stbdAzimuth output
function [portMP,portAzimuth,stbdMP,stbdAzimuth] = addNoise(PtThrust,...
    PtAzimuth,StThrust,StAzimuth,noiseLevel)
%Written By Anderson Lebbad on September 16, 2014
%Last Edited By:

%This function adds gaussian noise to the inputs for a particular particles
%model

portMP = normrnd(PtThrust, noiseLevel);
portAzimuth = normrnd(PtAzimuth, noiseLevel);
stbdMP = normrnd(StThrust, noiseLevel);
stbdAzimuth = normrnd(StAzimuth, noiseLevel);

end
